simulink model "design"  (R2025a)
settings: Solver=VariableStepAuto  StartTime=0.0  StopTime=10.0  RelTol=1e-3
InitFcn:
  | SSR=8;
undefined symbols (not defined in the file): xc7k325tffg900
libraries: hlsBasic x6, vmcUtilities x1
settings Model: Creator=admin  LastModifiedBy=robg
settings SolverCC: AlgebraicLoopSolver=TrustRegion
settings DataIOCC: ReturnWorkspaceOutputs=off
settings OptimizationCC: LifeSpan=inf
settings DebuggingCC: UnconnectedInputMsg=warning  UnconnectedOutputMsg=warning  UnconnectedLineMsg=warning  ArithmeticOperatorsInVariantConditions=warning
settings ModelReferenceCC: EnableRefExpFcnMdlSchedulingChecks=on
settings SFSimCC: SimUseLocalCustomCode=off  CustomCodeUndefinedFunction=UseInterfaceOnly
settings RTWCC: RTWUseLocalCustomCode=off  GPUComputeCapability=3.5
settings CodeAppCC: StateflowObjectComments=on

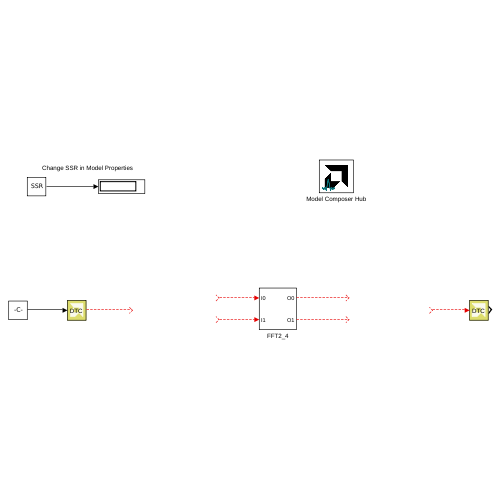
[thumbnail: Simulink's stored preview of the top-level diagram]
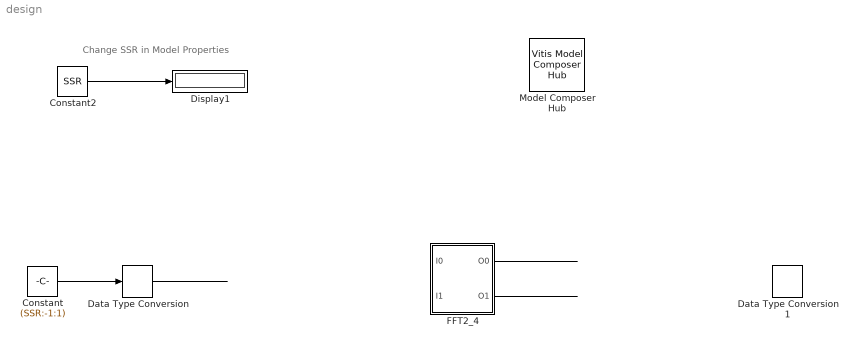
== system design ==
  note: Change SSR in Model Properties
  Constant : Constant  Value=(SSR:-1:1)  SampleTime=1
  Constant2 : Constant  Value=SSR  VectorParams1D=off  SampleTime=1
  Data Type Conversion : hlsBasic/Data Type Conversion  OutDataType=fixed  TypeExp=''  Signedness=Signed  WordLength=16  FractionalLength=8  RoundingMode=Truncation to minus infinity  OverflowMode=Wrap around
  Data Type Conversion1 : hlsBasic/Data Type Conversion  OutDataType=double  TypeExp=''  Signedness=Signed  WordLength=16  FractionalLength=0  RoundingMode=Truncation to minus infinity  OverflowMode=Wrap around
  Display1 : Display
  FFT2_4 : Subsystem
  Model Composer Hub : vmcUtilities/Vitis Model Composer Hub  Tag=genX  CodeGeneration=off  SubsystemName=Subsystem  StartColumn=1  NumberOfColumns=1  TargetDirectory=./code  exportDesign=off  analyzeDesign=off  validateDesignOnHw=off  ExportType=IP Catalog  IpVendor=xilinx.com  IpLibrary=hls  IpVersion=1.0  IpHWLanguage=Verilog  AieCompilerOptions={}  AieSimulatorOptions={}  CreateTestbench=off  TestbenchStackSize=10  RunRtlSim=off  RunCSim=off  RunAieSim=off  enableSimulationTimeout=on  enableGraphIterations=on  AieSimTimeout=50000  AieGraphIterations=-1  RunAieSimProfiling=off  LaunchVitisAnalyzer=off  PlotOutput=off  RunX86Sim=on  X86SimTimeout=10  GenHwImage=off  GenLibadfXo=off  GenHwValidationCode=off  PlatformType=Not Specified  HwSystemType=Baremetal  HwValidationTarget=hw  ProjDevice=Kintex-7 KC705 Evaluation Platform (xc7k325tffg900-2)  ProjDevicePart=xc7k325tffg900-2  SamplePeriod=-1  ClockFrequency=200  DataPathParallelism=1  xilinxfamily=Kintex7  part=xc7k325t  speed=-3  package=fbg676  directory=./netlist  testbench=off  incr_netlist=off  synthesis_tool=Vivado  clock_wrapper=Clock Enables  dbl_ovrd=According to Block Masks  dcm_input_clock_period=10  sysclk_period=10  simulink_period=1  eval_field=0  LogFileName=''  NThreads=4
  wires:
  Constant/1 -> Data Type Conversion/1
  Data Type Conversion/1 -> ?
  ? -> Data Type Conversion1/1
  FFT2_4/1(O0) -> ?
  FFT2_4/2(O1) -> ?
  ? -> FFT2_4/1(I0)
  ? -> FFT2_4/2(I1)
  Constant2/1 -> Display1/1

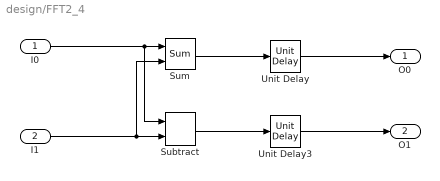
== system design/FFT2_4 ==
  I0 : Inport
  I1 : Inport  Port=2
  Subtract : hlsBasic/Subtract
  Sum : hlsBasic/Sum
  Unit Delay : hlsBasic/Unit Delay  InitialCondition=0
  Unit Delay3 : hlsBasic/Unit Delay  InitialCondition=0
  O0 : Outport
  O1 : Outport  Port=2
  wires:
  Sum/1 -> Unit Delay/1
  Unit Delay/1 -> O0/1
  Subtract/1 -> Unit Delay3/1
  Unit Delay3/1 -> O1/1
  I0/1 -> Subtract/1, Sum/1
  I1/1 -> Subtract/2, Sum/2
